simulink model "Adaptive_BS"  (R2021b)
settings: Solver=VariableStepAuto  StartTime=0.0  StopTime=15.0  MaxStep=1e-1  RelTol=1e1
values from neighbouring files (symbols this model uses):
  Kd = [100 0 0 0 0 0 0 150 0 0 0 0 ... (36 elements, 6x6)]    [ABS_workspace.mat]    (also in GuadagniControllore.m = diag([100 150 135 100 1 0.4]))
  l1 = 0.1273    [ABS_workspace.mat]
  l2 = -0.612    [ABS_workspace.mat]
  l3 = -0.5723    [ABS_workspace.mat]
  l4 = 0.1639    [ABS_workspace.mat]
  l5 = 0.1157    [ABS_workspace.mat]
  l6 = 0.0922    [ABS_workspace.mat]
  lambda = [10 0 0 0 0 0 0 90 0 0 0 0 ... (36 elements, 6x6)]    [ABS_workspace.mat]    (also in GuadagniControllore.m = diag([10 40 40 25 100 150]))
  m1 = 7.1    [ABS_workspace.mat]
  m2 = 12.7    [ABS_workspace.mat]
  m3 = 4.27    [ABS_workspace.mat]
  m4 = 2    [ABS_workspace.mat]
  m5 = 2    [ABS_workspace.mat]
  m6 = 0.365    [ABS_workspace.mat]
  q0 = [0 0 0 0 0 0]    [ABS_workspace.mat]
  r = 0.02    [ABS_workspace.mat]
undefined symbols (not defined in the file or in its folder): B, Spline
libraries: roblocks x3, robotcorelib x1, simulink x1
(part 5 of 5)

== matlab function Adaptive_BS/ABS control/parameters estimation ==
  data: Y input; dpi output; s input
function dpi = dyn_param(Y, s)
% Definisco una matrice definita positiva
R = diag([0.695 88 600 1200 1200 5000]);
% Calcolo la dinamica di stima dei parametri
dpi = inv(R) * Y' * s;
